simulink model "RS232ex2"  (Simulink 8.7)
settings: Solver=ode3  StartTime=0.0  StopTime=10.0  FixedStep=0.01  RelTol=1e-3
libraries: RS232 x6
settings Model: Creator=Leonardo  LastModifiedBy=Leonardo
settings DataIOCC: SignalLoggingSaveFormat=ModelDataLogs  SignalLoggingName=sigsOut
settings OptimizationCC: BlockReduction=off  BooleanDataType=off
settings DebuggingCC: SaveWithParameterizedLinksMsg=none  SignalResolutionControl=TryResolveAllWithWarning  MultiTaskDSMMsg=warning  MultiTaskCondExecSysMsg=none
settings HardwareCC: TargetUnknown=on
settings GRTTargetCC: GeneratePreprocessorConditionals=Use local settings  CombineOutputUpdateFcns=off  GRTInterface=on

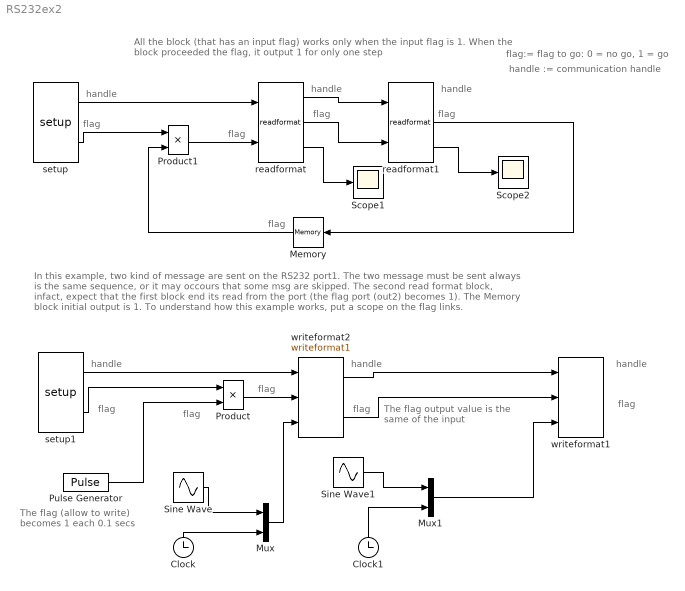
== system RS232ex2 ==
  note: In this example, two kind of message are sent on the RS232 port1. The two message must be sent always is
      | the same sequence, or it may occours that some msg are skipped. The second read format block, infact, expect
      | that the first block end its read from the port (the flag port (out2) becomes 1). The Memory block initial output is 1. To
      | understand how this example works, put a scope on the flag links.
  note: flag
  note: flag
  note: flag
  note: flag
  note: flag
  note: flag
  note: flag
  note: flag
  note: The flag (allow to write)
      | becomes 1 each 0.1 secs
  note: The flag output value
      | is the same of  the input
  note: flag
  note: flag:= flag to go: 0 = no go, 1 = go
  note: handle
  note: handle
  note: handle
  note: handle := communication handle
  note: handle
  note: handle
  note: handle
  note: flag
  note: All the block (that has an input flag) works only when the input flag is 1.
      | When the block proceeded the flag, it output 1 for only one step
  Clock : Clock
  Clock1 : Clock
  Memory : Memory  X0=1
  Mux : Mux  Inputs=2
  Mux1 : Mux  Inputs=2
  Product : Product  SaturateOnIntegerOverflow=on  OutDataTypeStr=Inherit: Same as first input
  Product1 : Product  SaturateOnIntegerOverflow=on  OutDataTypeStr=Inherit: Same as first input
  Pulse Generator : DiscretePulseGenerator  PulseType=Time based  Period=0.1  PulseWidth=10
  Scope1 : Scope
  Scope2 : Scope
  Sine Wave : Sin  SampleTime=0.01
  Sine Wave1 : Sin  Frequency=2  Phase=90  SampleTime=0.01
  readformat : RS232/readformat  fmtString=msg1;%f,%f;end  nCharTerm=4  sampTime=-1
  readformat1 : RS232/readformat  fmtString=msg2;%f,%f;end  nCharTerm=4  sampTime=-1
  setup : RS232/setup  port=COM2  baudrate=38400  databit=8  stopbit=1  parity=None
  setup1 : RS232/setup  port=COM3  baudrate=38400  databit=8  stopbit=1  parity=None
  writeformat1 : RS232/writeformat1  fmtString=msg2;%f,%f;end  sampTime=-1
  writeformat2 : RS232/writeformat1  fmtString=msg1;%f,%f;end  sampTime=-1
  wires:
  setup/1 -> readformat/1
  setup/2 -> Product1/1
  Memory/1 -> Product1/2
  setup1/1 -> writeformat2/1
  setup1/2 -> Product/1
  Clock/1 -> Mux/2
  Sine Wave/1 -> Mux/1
  Mux/1 -> writeformat2/3
  Pulse Generator/1 -> Product/2
  Product/1 -> writeformat2/2
  Product1/1 -> readformat/2
  readformat/3 -> Scope1/1
  readformat1/3 -> Scope2/1
  readformat/2 -> readformat1/2
  readformat/1 -> readformat1/1
  readformat1/2 -> Memory/1
  writeformat2/1 -> writeformat1/1
  Sine Wave1/1 -> Mux1/1
  Clock1/1 -> Mux1/2
  Mux1/1 -> writeformat1/3
  writeformat2/2 -> writeformat1/2
